simulink model "DC_power"  (R2023a)
settings: Solver=VariableStepAuto  StartTime=0.0  StopTime=5  MaxStep=1e-6  RelTol=1e-3
libraries: fl_lib x11, ee_lib x11, nesl_utility x11, simulink x3, spspowerguiLib x1
settings Model: Creator=MEHMET  LastModifiedBy=MEHMET
settings DebuggingCC: ParameterPrecisionLossMsg=none

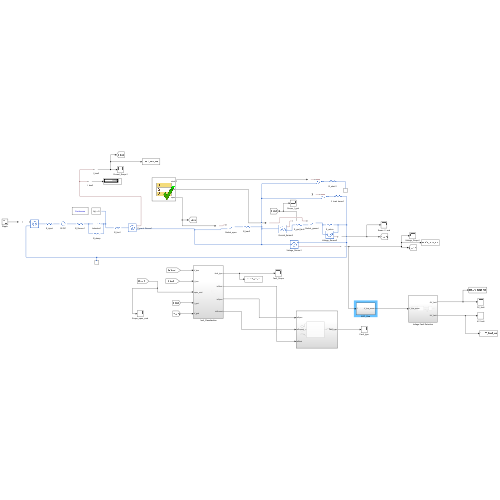
[thumbnail: Simulink's stored preview of the top-level diagram]
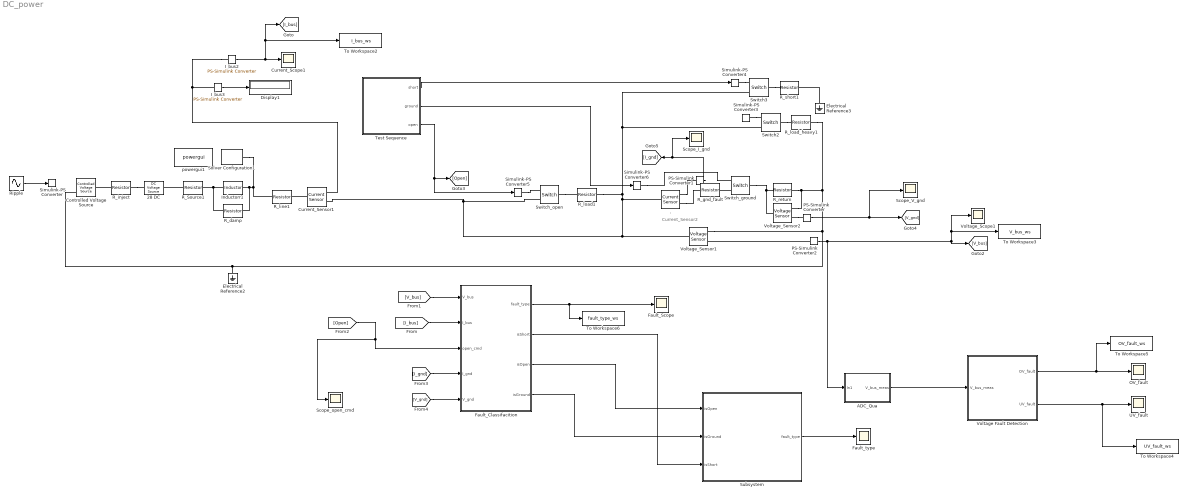
== system DC_power ==
  note: Current_Sensor2
  . : fl_lib/Electrical/Electrical Sensors/Current Sensor
  28 DC : ee_lib/Additional Components/SPICE Sources/DC Voltage Source  DC=28 V
  ADC_Qua : Subsystem
  Controlled Voltage Source : fl_lib/Electrical/Electrical Sources/Controlled Voltage Source
  Current_Scope1 : Scope
  Current_Sensor1 : fl_lib/Electrical/Electrical Sensors/Current Sensor
  Display1 : Display
  Electrical Reference2 : fl_lib/Electrical/Electrical Elements/Electrical Reference
  Electrical Reference3 : fl_lib/Electrical/Electrical Elements/Electrical Reference
  Fault_Classifacition : Subsystem
  Fault_Scope : Scope
  Fault_type : Scope
  I_bus2 : nesl_utility/PS-Simulink Converter  PhysicalDomain=network_engine_domain  SubClassName=ps_output  LeftPortType=input  RightPortType=output  PseudoPeriodic=off  Frequencies=[]  VectorFormat=inherit  Unit=inherit  AffineConversion=off
  I_bus3 : nesl_utility/PS-Simulink Converter  PhysicalDomain=network_engine_domain  SubClassName=ps_output  LeftPortType=input  RightPortType=output  PseudoPeriodic=off  Frequencies=[]  VectorFormat=inherit  Unit=inherit  AffineConversion=off
  Inductorr1 : ee_lib/Passive/Inductor  l=20e-6 H  enable_L_tol=ee.enum.toleranceApplication.none  L_tol=20  tol_distribution=ee.enum.toleranceDistribution.uniform  nSigma=4  r=0 Ohm  g=1e-9 1/Ohm  enable_operating_limits=ee.enum.enable.no  operating_limit_action=ee.enum.passive.reportOpLim.warn  max_working_current=1 A  power_rating=1 W  enable_faults=ee.enum.enable.no  fault_action=simscape.enum.assert.action.none  lambdaPercent=50  k_faulted=0.9999  turnsShort=ee.enum.passive.inductor.turnsShortOption.no  openCct=ee.enum.enable.no  groundShort=ee.enum.passive.inductor.groundShortOption.no  groundShortG=0 1/Ohm  tau_fault=1e-3 s  fault_trigger=ee.enum.faults.faultTrigger.temporal  t_fault=1 s  max_permissible_voltage=100 V  n_fail_on_voltage=1  max_permissible_current=1 A  t_fail_on_current=1 s  i_L_specify=off  i_L_priority=High  i_L=0 A  i_L_nominal_specify=off  i_L_nominal_unit=A  i_L_nominal_value=1
  OV_fault : Scope
  PS-Simulink Converter : nesl_utility/PS-Simulink Converter  PhysicalDomain=network_engine_domain  SubClassName=ps_output  LeftPortType=input  RightPortType=output  PseudoPeriodic=off  Frequencies=[]  VectorFormat=inherit  Unit=inherit  AffineConversion=off
  PS-Simulink Converter1 : nesl_utility/PS-Simulink Converter  PhysicalDomain=network_engine_domain  SubClassName=ps_output  LeftPortType=input  RightPortType=output  PseudoPeriodic=off  Frequencies=[]  VectorFormat=inherit  Unit=inherit  AffineConversion=off
  PS-Simulink Converter2 : nesl_utility/PS-Simulink Converter  PhysicalDomain=network_engine_domain  SubClassName=ps_output  LeftPortType=input  RightPortType=output  PseudoPeriodic=off  Frequencies=[]  VectorFormat=inherit  Unit=inherit  AffineConversion=off
  R_Source1 : ee_lib/Passive/Resistor  R=0.1 Ohm  enable_R_tol=ee.enum.toleranceApplication.none  R_tol=5  tol_distribution=ee.enum.toleranceDistribution.uniform  nSigma=4  enable_operating_limits=ee.enum.enable.no  operating_limit_action=ee.enum.passive.reportOpLim.warn  power_rating=1 W  max_working_voltage=100 V  enable_faults=ee.enum.enable.no  fault_action=simscape.enum.assert.action.none  R_faulted=inf Ohm  fault_trigger=ee.enum.faults.faultTrigger.temporal  t_fault=1 s  max_permissible_current=1 A  t_fail_on_current=1 s  noise_mode=ee.enum.sources.noise.Disabled  Tdevice=25 degC  sample_time=1e-3 s  repeatability=ee.enum.ic.repeatability.notRepeatable  user_seed=0  auto_seed=3890346746  power_derating_T1=70 degC  power_derating_T2=155 degC  operating_temperature_range_vec=[-50, 150] degC  alpha=3.93e-3 1/K  Tmeas=25 degC  thermal_mass=100 J/K  temperature_specify=off  temperature_priority=High  temperature=298.15 K  temperature_nominal_specify=off  temperature_nominal_unit=K  temperature_nominal_value=1
  R_damp : ee_lib/Passive/Resistor  R=10 Ohm  enable_R_tol=ee.enum.toleranceApplication.none  R_tol=5  tol_distribution=ee.enum.toleranceDistribution.uniform  nSigma=4  enable_operating_limits=ee.enum.enable.no  operating_limit_action=ee.enum.passive.reportOpLim.warn  power_rating=1 W  max_working_voltage=100 V  enable_faults=ee.enum.enable.no  fault_action=simscape.enum.assert.action.none  R_faulted=inf Ohm  fault_trigger=ee.enum.faults.faultTrigger.temporal  t_fault=1 s  max_permissible_current=1 A  t_fail_on_current=1 s  noise_mode=ee.enum.sources.noise.Disabled  Tdevice=25 degC  sample_time=1e-3 s  repeatability=ee.enum.ic.repeatability.notRepeatable  user_seed=0  auto_seed=3922919431  power_derating_T1=70 degC  power_derating_T2=155 degC  operating_temperature_range_vec=[-50, 150] degC  alpha=3.93e-3 1/K  Tmeas=25 degC  thermal_mass=100 J/K  temperature_specify=off  temperature_priority=High  temperature=298.15 K  temperature_nominal_specify=off  temperature_nominal_unit=K  temperature_nominal_value=1
  R_gnd_fault : ee_lib/Passive/Resistor  R=5 Ohm  enable_R_tol=ee.enum.toleranceApplication.none  R_tol=5  tol_distribution=ee.enum.toleranceDistribution.uniform  nSigma=4  enable_operating_limits=ee.enum.enable.no  operating_limit_action=ee.enum.passive.reportOpLim.warn  power_rating=1 W  max_working_voltage=100 V  enable_faults=ee.enum.enable.no  fault_action=simscape.enum.assert.action.none  R_faulted=inf Ohm  fault_trigger=ee.enum.faults.faultTrigger.temporal  t_fault=1 s  max_permissible_current=1 A  t_fail_on_current=1 s  noise_mode=ee.enum.sources.noise.Disabled  Tdevice=25 degC  sample_time=1e-3 s  repeatability=ee.enum.ic.repeatability.notRepeatable  user_seed=0  auto_seed=1196140742  power_derating_T1=70 degC  power_derating_T2=155 degC  operating_temperature_range_vec=[-50, 150] degC  alpha=3.93e-3 1/K  Tmeas=25 degC  thermal_mass=100 J/K  temperature_specify=off  temperature_priority=High  temperature=298.15 K  temperature_nominal_specify=off  temperature_nominal_unit=K  temperature_nominal_value=1
  R_inject : ee_lib/Passive/Resistor  R=0.1 Ohm  enable_R_tol=ee.enum.toleranceApplication.none  R_tol=5  tol_distribution=ee.enum.toleranceDistribution.uniform  nSigma=4  enable_operating_limits=ee.enum.enable.no  operating_limit_action=ee.enum.passive.reportOpLim.warn  power_rating=1 W  max_working_voltage=100 V  enable_faults=ee.enum.enable.no  fault_action=simscape.enum.assert.action.none  R_faulted=inf Ohm  fault_trigger=ee.enum.faults.faultTrigger.temporal  t_fault=1 s  max_permissible_current=1 A  t_fail_on_current=1 s  noise_mode=ee.enum.sources.noise.Disabled  Tdevice=25 degC  sample_time=1e-3 s  repeatability=ee.enum.ic.repeatability.notRepeatable  user_seed=0  auto_seed=3499211588  power_derating_T1=70 degC  power_derating_T2=155 degC  operating_temperature_range_vec=[-50, 150] degC  alpha=3.93e-3 1/K  Tmeas=25 degC  thermal_mass=100 J/K  temperature_specify=off  temperature_priority=High  temperature=298.15 K  temperature_nominal_specify=off  temperature_nominal_unit=K  temperature_nominal_value=1
  R_line1 : ee_lib/Passive/Resistor  R=0.2 Ohm  enable_R_tol=ee.enum.toleranceApplication.none  R_tol=5  tol_distribution=ee.enum.toleranceDistribution.uniform  nSigma=4  enable_operating_limits=ee.enum.enable.no  operating_limit_action=ee.enum.passive.reportOpLim.warn  power_rating=1 W  max_working_voltage=100 V  enable_faults=ee.enum.enable.no  fault_action=simscape.enum.assert.action.none  R_faulted=inf Ohm  fault_trigger=ee.enum.faults.faultTrigger.temporal  t_fault=1 s  max_permissible_current=1 A  t_fail_on_current=1 s  noise_mode=ee.enum.sources.noise.Disabled  Tdevice=25 degC  sample_time=1e-3 s  repeatability=ee.enum.ic.repeatability.notRepeatable  user_seed=0  auto_seed=545404223  power_derating_T1=70 degC  power_derating_T2=155 degC  operating_temperature_range_vec=[-50, 150] degC  alpha=3.93e-3 1/K  Tmeas=25 degC  thermal_mass=100 J/K  temperature_specify=off  temperature_priority=High  temperature=298.15 K  temperature_nominal_specify=off  temperature_nominal_unit=K  temperature_nominal_value=1
  R_load1 : ee_lib/Passive/Resistor  R=56 Ohm  enable_R_tol=ee.enum.toleranceApplication.none  R_tol=5  tol_distribution=ee.enum.toleranceDistribution.uniform  nSigma=4  enable_operating_limits=ee.enum.enable.no  operating_limit_action=ee.enum.passive.reportOpLim.warn  power_rating=1 W  max_working_voltage=100 V  enable_faults=ee.enum.enable.no  fault_action=simscape.enum.assert.action.none  R_faulted=inf Ohm  fault_trigger=ee.enum.faults.faultTrigger.temporal  t_fault=1 s  max_permissible_current=1 A  t_fail_on_current=1 s  noise_mode=ee.enum.sources.noise.Disabled  Tdevice=25 degC  sample_time=1e-3 s  repeatability=ee.enum.ic.repeatability.notRepeatable  user_seed=0  auto_seed=3499211588  power_derating_T1=70 degC  power_derating_T2=155 degC  operating_temperature_range_vec=[-50, 150] degC  alpha=3.93e-3 1/K  Tmeas=25 degC  thermal_mass=100 J/K  temperature_specify=off  temperature_priority=High  temperature=298.15 K  temperature_nominal_specify=off  temperature_nominal_unit=K  temperature_nominal_value=1
  R_load_heavy1 : ee_lib/Passive/Resistor  R=14 Ohm  enable_R_tol=ee.enum.toleranceApplication.none  R_tol=5  tol_distribution=ee.enum.toleranceDistribution.uniform  nSigma=4  enable_operating_limits=ee.enum.enable.no  operating_limit_action=ee.enum.passive.reportOpLim.warn  power_rating=1 W  max_working_voltage=100 V  enable_faults=ee.enum.enable.no  fault_action=simscape.enum.assert.action.none  R_faulted=inf Ohm  fault_trigger=ee.enum.faults.faultTrigger.temporal  t_fault=1 s  max_permissible_current=1 A  t_fail_on_current=1 s  noise_mode=ee.enum.sources.noise.Disabled  Tdevice=25 degC  sample_time=1e-3 s  repeatability=ee.enum.ic.repeatability.notRepeatable  user_seed=0  auto_seed=2715962282  power_derating_T1=70 degC  power_derating_T2=155 degC  operating_temperature_range_vec=[-50, 150] degC  alpha=3.93e-3 1/K  Tmeas=25 degC  thermal_mass=100 J/K  temperature_specify=off  temperature_priority=High  temperature=298.15 K  temperature_nominal_specify=off  temperature_nominal_unit=K  temperature_nominal_value=1
  R_return : ee_lib/Passive/Resistor  R=0.05 Ohm  enable_R_tol=ee.enum.toleranceApplication.none  R_tol=5  tol_distribution=ee.enum.toleranceDistribution.uniform  nSigma=4  enable_operating_limits=ee.enum.enable.no  operating_limit_action=ee.enum.passive.reportOpLim.warn  power_rating=1 W  max_working_voltage=100 V  enable_faults=ee.enum.enable.no  fault_action=simscape.enum.assert.action.none  R_faulted=inf Ohm  fault_trigger=ee.enum.faults.faultTrigger.temporal  t_fault=1 s  max_permissible_current=1 A  t_fail_on_current=1 s  noise_mode=ee.enum.sources.noise.Disabled  Tdevice=25 degC  sample_time=1e-3 s  repeatability=ee.enum.ic.repeatability.notRepeatable  user_seed=0  auto_seed=3499211588  power_derating_T1=70 degC  power_derating_T2=155 degC  operating_temperature_range_vec=[-50, 150] degC  alpha=3.93e-3 1/K  Tmeas=25 degC  thermal_mass=100 J/K  temperature_specify=off  temperature_priority=High  temperature=298.15 K  temperature_nominal_specify=off  temperature_nominal_unit=K  temperature_nominal_value=1
  R_short1 : ee_lib/Passive/Resistor  R=0.001 Ohm  enable_R_tol=ee.enum.toleranceApplication.none  R_tol=5  tol_distribution=ee.enum.toleranceDistribution.uniform  nSigma=4  enable_operating_limits=ee.enum.enable.no  operating_limit_action=ee.enum.passive.reportOpLim.warn  power_rating=1 W  max_working_voltage=100 V  enable_faults=ee.enum.enable.no  fault_action=simscape.enum.assert.action.none  R_faulted=inf Ohm  fault_trigger=ee.enum.faults.faultTrigger.temporal  t_fault=1 s  max_permissible_current=1 A  t_fail_on_current=1 s  noise_mode=ee.enum.sources.noise.Disabled  Tdevice=25 degC  sample_time=1e-3 s  repeatability=ee.enum.ic.repeatability.notRepeatable  user_seed=0  auto_seed=418932850  power_derating_T1=70 degC  power_derating_T2=155 degC  operating_temperature_range_vec=[-50, 150] degC  alpha=3.93e-3 1/K  Tmeas=25 degC  thermal_mass=100 J/K  temperature_specify=off  temperature_priority=High  temperature=298.15 K  temperature_nominal_specify=off  temperature_nominal_unit=K  temperature_nominal_value=1
  Ripple : Sin  Amplitude=0.3  Frequency=1000  SampleTime=0
  Scope_I_gnd : Scope
  Scope_V_gnd : Scope
  Scope_open_cmd : Scope
  Simulink-PS Converter{,3..6} (5 alike) : nesl_utility/Simulink-PS Converter  PhysicalDomain=network_engine_domain  SubClassName=ps_input  LeftPortType=input  RightPortType=output  PseudoPeriodic=off  Frequencies=[]  NoiseDistribution=none  NoiseParameters=[]  Unit=1  AffineConversion=off  FilteringAndDerivatives=provide  SimscapeFilterOrder=1  InputFilterTimeConstant=0.001  UdotUserProvided=0
  Solver Configuration1 : nesl_utility/Solver Configuration  PhysicalDomain=network_engine_domain  SubClassName=solver  LeftPortType=input  RightPortType=generic  Tones=[]  Harmonics=[]  SimulateNoise=off  Profile=off  UseLocalSampling=off  EnableSwitchedLinearOptims=on  FrequencyDomain=off  UseCCode=off  RelTol=0.001  AbsTol=0.001  MinStep=1e-09  ToWorkspace=off  RevertToSquareIcSolve=off  NumHomotopyIterations=100  PhasorMode=off  PhasorModeNumHarmonics=1  ConsistencySolver=NEWTON_XTOL_AFTER_FTOL  IndexReductionMethod=DerivativeReplacement  DoDC=off  ResidualTolerance=1e-09  ConsistencyTolSource=GLOBAL  ConsistencyAbsTol=0.001  ConsistencyRelTol=0.001  ConsistencyTolFactor=0.001  UseLocalSolver=off  LocalSolverChoice=NE_BACKWARD_EULER_ADVANCER  ResolveIndetEquations=on  FunctionEvalNumThread=1  LocalSolverSampleTime=0.001  DoFixedCost=off  MaxNonlinIter=3  MaxModeIter=2  ComputeImpulses=off  ImpulseIterations=2  LinearAlgebra=auto  LinearAlgebraNumThread=0  EquationFormulation=NE_TIME_EF  DelaysMemoryBudget=1024  AutomaticFiltering=on  FilteringTimeConstant=0.001  PartitionStorageMethod=AS_NEEDED  PartitionMemoryBudget=1024  PartitionMethod=ROBUST
  Subsystem : Subsystem
  Switch2 : fl_lib/Electrical/Electrical Elements/Switch  R_closed=0.01 Ohm  G_open=1e-8 1/Ohm  Threshold=0.5  i_specify=off  i_priority=None  i=0 A  i_nominal_specify=off  i_nominal_unit=A  i_nominal_value=1  v_specify=off  v_priority=None  v=0 V  v_nominal_specify=off  v_nominal_unit=V  v_nominal_value=1
  Switch3 : fl_lib/Electrical/Electrical Elements/Switch  R_closed=0.01 Ohm  G_open=1e-8 1/Ohm  Threshold=0.5  i_specify=off  i_priority=None  i=0 A  i_nominal_specify=off  i_nominal_unit=A  i_nominal_value=1  v_specify=off  v_priority=None  v=0 V  v_nominal_specify=off  v_nominal_unit=V  v_nominal_value=1
  Switch_ground : fl_lib/Electrical/Electrical Elements/Switch  R_closed=0.01 Ohm  G_open=1e-8 1/Ohm  Threshold=0.5  i_specify=off  i_priority=None  i=0 A  i_nominal_specify=off  i_nominal_unit=A  i_nominal_value=1  v_specify=off  v_priority=None  v=0 V  v_nominal_specify=off  v_nominal_unit=V  v_nominal_value=1
  Switch_open : fl_lib/Electrical/Electrical Elements/Switch  R_closed=0.01 Ohm  G_open=1e-8 1/Ohm  Threshold=0.5  i_specify=off  i_priority=None  i=0 A  i_nominal_specify=off  i_nominal_unit=A  i_nominal_value=1  v_specify=off  v_priority=None  v=0 V  v_nominal_specify=off  v_nominal_unit=V  v_nominal_value=1
  Test Sequence : Test Sequence  TreatAsAtomicUnit=on
  To Workspace2 : ToWorkspace  VariableName=I_bus_ws  SaveFormat=Structure With Time  SampleTime=-1
  To Workspace3 : ToWorkspace  VariableName=V_bus_ws  SaveFormat=Structure With Time  SampleTime=-1
      settings: MaxDataPoints=Inf
  To Workspace4 : ToWorkspace  VariableName=UV_fault_ws  SaveFormat=Timeseries  SampleTime=-1
  To Workspace5 : ToWorkspace  VariableName=OV_fault_ws  SaveFormat=Timeseries  SampleTime=-1
  To Workspace6 : ToWorkspace  VariableName=fault_type_ws  SaveFormat=Timeseries  SampleTime=-1
  UV_fault : Scope
  Voltage Fault Detection : Subsystem
  Voltage_Scope1 : Scope
  Voltage_Sensor1 : fl_lib/Electrical/Electrical Sensors/Voltage Sensor
  Voltage_Sensor2 : fl_lib/Electrical/Electrical Sensors/Voltage Sensor
  powergui1 : spspowerguiLib/powergui  Priority=1  SimulationMode=Continuous  SampleTime=50e-6  frequency=60  Iterations=50  frequencyindice=60  Pbase=100e6  ErrMax=1e-4  UnitsV=kV  UnitsW=MW  buscounter=0  FunctionMessages=off  echomessages=off  EnableUseOfTLC=off  CurrentSourceSwitches=off  DisableSnubberDevices=off  DisableRonSwitches=off  DisableVfSwitches=off  DisplayEquations=off  AutomaticDiscreteSolvers=off  SolverType=Tustin/Backward Euler (TBE)  Interpol=off  ExternalGateDelay=off  methode=off  Ts=100  x0status=blocks  SPID=on  SwTol=0  HookPort=off  NonlinearTolerance=1e-4  nMaxIteration=100  ContinueOnMaxIteration=off  RestoreLinks=warning  ResistiveCurrentMeasurement=off  Frange=[0:2:500]  Ylog=off  Xlog=on  ShowGrid=off  save=off  variable=ZData  structure=0  ZoomFFT=off  StartTime=0.0  cycles=1  DisplayStyle=1  fundamental=60  FreqAxis=off  MaxFrequency=1000  frequencyindicesteady=1  RmsSteady=1  display=off
  wires:
  I_bus3/1 -> Display1/1
  I_bus2/1 -> To Workspace2/1, [I_bus], Current_Scope1/1
  Test Sequence/1(short) -> Simulink-PS Converter4/1
  Test Sequence/2(ground) -> Simulink-PS Converter6/1
  Test Sequence/3(open) -> Simulink-PS Converter5/1, [Open]
  Fault_Classifacition/1(fault_type) -> To Workspace6/1, Fault_Scope/1
  [V_bus] -> Fault_Classifacition/1(V_bus)
  [I_bus] -> Fault_Classifacition/2(I_bus)
  [Open] -> Fault_Classifacition/3(open_cmd), Scope_open_cmd/1
  PS-Simulink Converter/1 -> Scope_V_gnd/1, [V_gnd]
  PS-Simulink Converter1/1 -> Scope_I_gnd/1, [I_gnd]
  [I_gnd] -> Fault_Classifacition/4(I_gnd)
  [V_gnd] -> Fault_Classifacition/5(V_gnd)
  ADC_Qua/1(V_bus_meas) -> Voltage Fault Detection/1(V_bus_meas)
  Voltage Fault Detection/1(OV_fault) -> To Workspace5/1, OV_fault/1
  Fault_Classifacition/3(isOpen) -> Subsystem/1(isOpen)
  Fault_Classifacition/4(isGround) -> Subsystem/2(isGround)
  Fault_Classifacition/2(isShort) -> Subsystem/3(isShort)
  Subsystem/1(fault_type) -> Fault_type/1
  Voltage Fault Detection/2(UV_fault) -> To Workspace4/1, UV_fault/1
  PS-Simulink Converter2/1 -> [V_bus], To Workspace3/1, Voltage_Scope1/1, ADC_Qua/1(In1)
  Ripple/1 -> Simulink-PS Converter/1
  connections:
  R_line1/LConn1 -- Solver Configuration1/RConn1 -- R_damp/RConn1 -- Inductorr1/RConn1
  I_bus2/LConn1 -- Current_Sensor1/RConn1 -- I_bus3/LConn1
  Switch2/LConn1 -- R_load_heavy1/LConn1
  Switch3/LConn1 -- R_short1/LConn1
  Simulink-PS Converter4/RConn1 -- Switch3/RConn1
  Simulink-PS Converter3/RConn1 -- Switch2/RConn1
  Electrical Reference3/LConn1 -- R_short1/RConn1
  PS-Simulink Converter2/LConn1 -- Voltage_Sensor1/RConn1
  Inductorr1/LConn1 -- R_damp/LConn1 -- R_Source1/RConn1
  Current_Sensor1/LConn1 -- R_line1/RConn1
  Voltage_Sensor2/RConn2 -- R_return/RConn1 -- R_load_heavy1/RConn1 -- Electrical Reference2/LConn1 -- Controlled Voltage Source/RConn2 -- Voltage_Sensor1/RConn2
  Voltage_Sensor2/RConn1 -- PS-Simulink Converter/LConn1
  ./RConn1 -- PS-Simulink Converter1/LConn1
  Switch_open/LConn1 -- R_load1/LConn1
  Simulink-PS Converter5/RConn1 -- Switch_open/RConn1
  Voltage_Sensor2/LConn1 -- Switch_ground/LConn1 -- R_return/LConn1
  ./RConn2 -- R_gnd_fault/LConn1
  Simulink-PS Converter6/RConn1 -- Switch_ground/RConn1
  Switch_ground/RConn2 -- R_gnd_fault/RConn1
  R_Source1/LConn1 -- 28 DC/LConn1
  R_inject/RConn1 -- 28 DC/RConn1
  R_inject/LConn1 -- Controlled Voltage Source/LConn1
  Current_Sensor1/RConn2 -- Switch_open/RConn2 -- R_load1/RConn1 -- Switch3/RConn2 -- Switch2/RConn2 -- ./LConn1 -- Voltage_Sensor1/LConn1

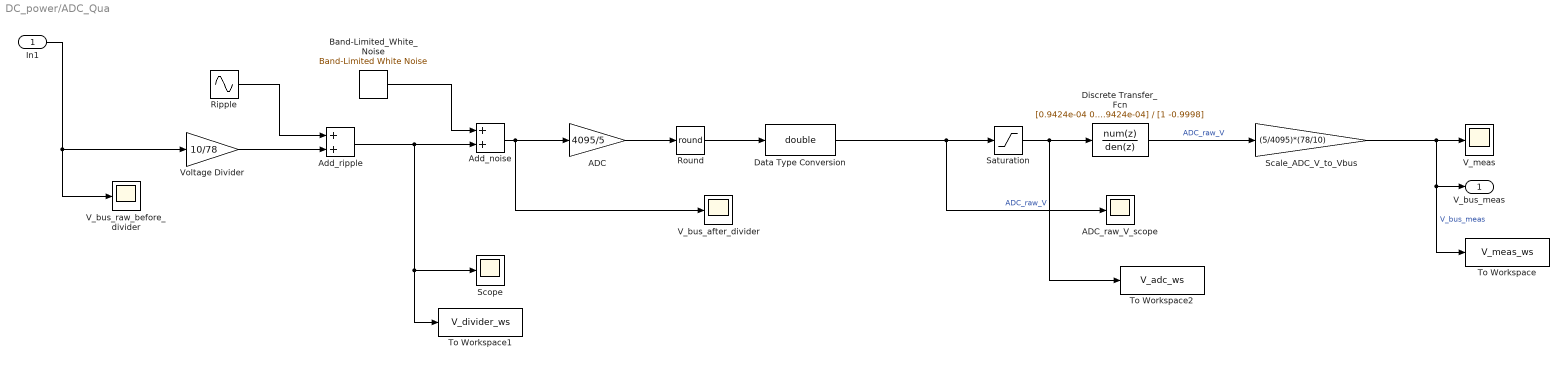
== system DC_power/ADC_Qua ==
  In1 : Inport
  ADC : Gain  Gain=4095/5
  ADC_raw_V_scope : Scope
  Add_noise : Sum
  Add_ripple : Sum
  Band-Limited_White_Noise : simulink/Sources/Band-Limited White Noise  Cov=1e-12  Ts=1e-5  seed=[123]
  Data Type Conversion : DataTypeConversion  OutDataTypeStr=double  SaturateOnIntegerOverflow=off  RndMeth=Floor
  Discrete Transfer_Fcn : DiscreteTransferFcn  Numerator=[0.9424e-04 0.9424e-04]  Denominator=[1 -0.9998]  SampleTime=1e-6
  Ripple : Sin  SampleTime=0
  Round : Rounding  Operator=round
  Saturation : Saturate  UpperLimit=4095  LowerLimit=0  ZeroCross=off
  Scale_ADC_V_to_Vbus : Gain  Gain=(5/4095)*(78/10)
  Scope : Scope
  To Workspace : ToWorkspace  VariableName=V_meas_ws  SaveFormat=Timeseries  SampleTime=-1
  To Workspace1 : ToWorkspace  VariableName=V_divider_ws  SaveFormat=Timeseries  SampleTime=-1
  To Workspace2 : ToWorkspace  VariableName=V_adc_ws  SaveFormat=Timeseries  SampleTime=-1
  V_bus_after_divider : Scope
  V_bus_raw_before_divider : Scope
  V_meas : Scope
  Voltage Divider : Gain  Gain=10/78
  V_bus_meas : Outport
  wires:
  In1/1 -> V_bus_raw_before_divider/1, Voltage Divider/1
  Scale_ADC_V_to_Vbus/1 -> To Workspace/1, V_bus_meas/1, V_meas/1  "V_bus_meas"
  Voltage Divider/1 -> Add_ripple/2
  Add_ripple/1 -> To Workspace1/1, Scope/1, Add_noise/2
  Saturation/1 -> To Workspace2/1, Discrete Transfer_Fcn/1
  Add_noise/1 -> V_bus_after_divider/1, ADC/1
  Round/1 -> Data Type Conversion/1
  Data Type Conversion/1 -> Saturation/1, ADC_raw_V_scope/1  "ADC_raw_V"
  Discrete Transfer_Fcn/1 -> Scale_ADC_V_to_Vbus/1  "ADC_raw_V"
  ADC/1 -> Round/1
  Band-Limited_White_Noise/1 -> Add_noise/1
  Ripple/1 -> Add_ripple/1

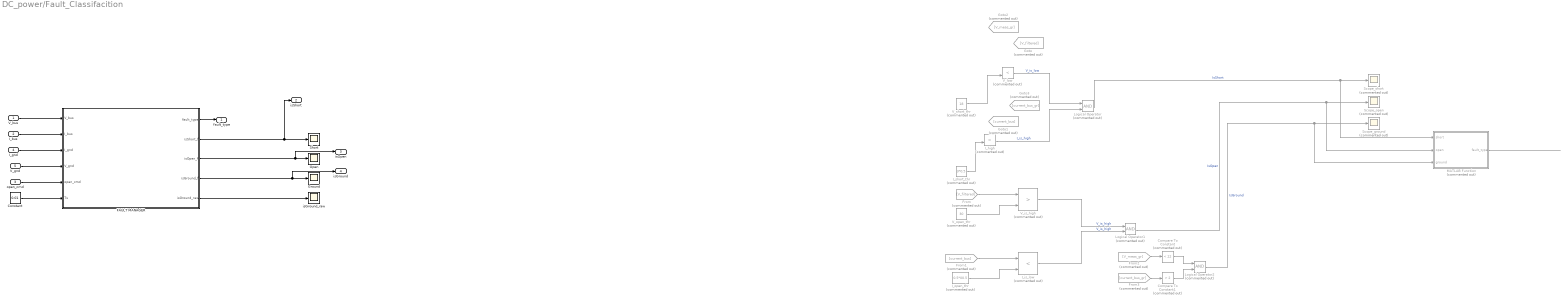
== system DC_power/Fault_Classifacition ==
  V_bus : Inport
  I_bus : Inport  Port=2
  open_cmd : Inport  Port=3
  I_gnd : Inport  Port=4
  V_gnd : Inport  Port=5
  Compare To Constant : simulink/Logic and Bit Operations/Compare To Constant  Commented=on  relop=<  const=22  OutDataTypeStr=boolean  ZeroCross=off
  Compare To Constant1 : simulink/Logic and Bit Operations/Compare To Constant  Commented=on  relop=>  const=2  OutDataTypeStr=boolean  ZeroCross=off
  Constant : Constant  Value=0.01
  FAULT MANAGER : MATLAB Function  TreatAsAtomicUnit=on
  From : From  Commented=on  GotoTag=V_filtered
  From1 : From  Commented=on  GotoTag=current_bus
  From2 : From  Commented=on  GotoTag=V_meas_gr
  From3 : From  Commented=on  GotoTag=current_bus_gr
  Goto : Goto  Commented=on  GotoTag=V_filtered
  Goto1 : Goto  Commented=on  GotoTag=current_bus
  Goto2 : Goto  Commented=on  GotoTag=V_meas_gr
  Goto3 : Goto  Commented=on  GotoTag=current_bus_gr
  Ground : Scope
  I_high : RelationalOperator  Commented=on  Operator=>  OutDataTypeStr=boolean  RndMeth=Simplest  InputSameDT=off
  I_is_low : RelationalOperator  Commented=on  Operator=<  OutDataTypeStr=boolean  RndMeth=Simplest  InputSameDT=off
  I_open_thr : Constant  Commented=on  Value=0.5*00.5
  I_short_thr : Constant  Commented=on  Value=3*0.5
  Logical Operator : Logic  Commented=on  AllPortsSameDT=off  OutDataTypeStr=boolean
  Logical Operator1 : Logic  Commented=on  AllPortsSameDT=off  OutDataTypeStr=boolean
  Logical Operator2 : Logic  Commented=on  AllPortsSameDT=off  OutDataTypeStr=boolean
  MATLAB Function : MATLAB Function  Commented=on  TreatAsAtomicUnit=on
  Open : Scope
  Scope_ground : Scope  Commented=on
  Scope_open : Scope  Commented=on
  Scope_short : Scope  Commented=on
  Short : Scope
  V_is_high : RelationalOperator  Commented=on  Operator=>  OutDataTypeStr=boolean  RndMeth=Simplest  InputSameDT=off
  V_low : RelationalOperator  Commented=on  Operator=<  OutDataTypeStr=boolean  RndMeth=Simplest  InputSameDT=off
  V_open_thr : Constant  Commented=on  Value=30
  V_short_thr : Constant  Commented=on  Value=18
  isGround_raw : Scope
  fault_type : Outport
  isShort : Outport  Port=2
  isOpen : Outport  Port=3
  isGround : Outport  Port=4
  wires:
  ? -> Goto2/1, Goto/1, V_low/1
  V_short_thr/1 -> V_low/2
  V_low/1 -> Logical Operator/1  "V_is_low"
  ? -> Goto3/1, Goto1/1, I_high/1
  I_short_thr/1 -> I_high/2
  I_high/1 -> Logical Operator/2  "I_is_high"
  Logical Operator/1 -> MATLAB Function/1(short), Scope_short/1  "IsShort"
  From/1 -> V_is_high/1
  V_open_thr/1 -> V_is_high/2
  V_is_high/1 -> Logical Operator1/1  "V_is_high"
  I_is_low/1 -> Logical Operator1/2  "V_is_high"
  I_open_thr/1 -> I_is_low/2
  From1/1 -> I_is_low/1
  Logical Operator1/1 -> MATLAB Function/2(open), Scope_open/1  "IsOpen"
  MATLAB Function/1(fault_type) -> ?
  From2/1 -> Compare To Constant/1
  From3/1 -> Compare To Constant1/1
  Compare To Constant/1 -> Logical Operator2/1
  Compare To Constant1/1 -> Logical Operator2/2
  Logical Operator2/1 -> MATLAB Function/3(ground), Scope_ground/1  "IsGround"
  V_bus/1 -> FAULT MANAGER/1(V_bus)
  I_bus/1 -> FAULT MANAGER/2(I_bus)
  Constant/1 -> FAULT MANAGER/6(Ts)
  FAULT MANAGER/2(isShort_f) -> isShort/1, Short/1
  FAULT MANAGER/3(isOpen_f) -> isOpen/1, Open/1
  FAULT MANAGER/4(isGround_f) -> isGround/1, Ground/1
  FAULT MANAGER/1(fault_type) -> fault_type/1
  open_cmd/1 -> FAULT MANAGER/5(open_cmd)
  I_gnd/1 -> FAULT MANAGER/3(I_gnd)
  V_gnd/1 -> FAULT MANAGER/4(V_gnd)
  FAULT MANAGER/5(isGround_raw) -> isGround_raw/1

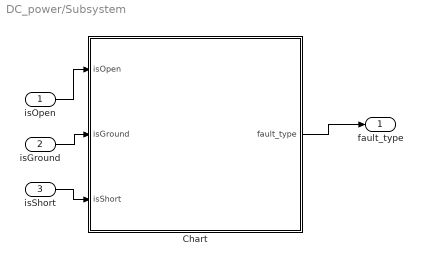
== system DC_power/Subsystem ==
  isOpen : Inport
  isGround : Inport  Port=2
  isShort : Inport  Port=3
  Chart : Stateflow chart  TreatAsAtomicUnit=on
  fault_type : Outport
  wires:
  isShort/1 -> Chart/3(isShort)
  isGround/1 -> Chart/2(isGround)
  isOpen/1 -> Chart/1(isOpen)
  Chart/1(fault_type) -> fault_type/1

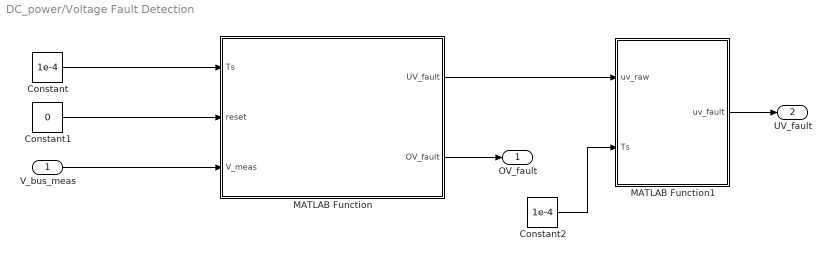
== system DC_power/Voltage Fault Detection ==
  V_bus_meas : Inport
  Constant : Constant  Value=1e-4
  Constant1 : Constant  Value=0
  Constant2 : Constant  Value=1e-4
  MATLAB Function : MATLAB Function  TreatAsAtomicUnit=on
  MATLAB Function1 : MATLAB Function  TreatAsAtomicUnit=on
  OV_fault : Outport
  UV_fault : Outport  Port=2
  wires:
  Constant/1 -> MATLAB Function/1(Ts)
  Constant1/1 -> MATLAB Function/2(reset)
  MATLAB Function/1(UV_fault) -> MATLAB Function1/1(uv_raw)
  MATLAB Function/2(OV_fault) -> OV_fault/1
  Constant2/1 -> MATLAB Function1/2(Ts)
  MATLAB Function1/1(uv_fault) -> UV_fault/1
  V_bus_meas/1 -> MATLAB Function/3(V_meas)

== matlab function DC_power/Fault_Classifacition/FAULT MANAGER ==
  settings: updateMethod=DISCRETE
  data: V_bus input; fault_type output; I_bus input; I_gnd input; V_gnd input; open_cmd input; Ts input; isShort_f output boolean size=1; isOpen_f output boolean size=1; isGround_f output boolean size=1; isGround_raw output boolean size=1
function [fault_type, isShort_f, isOpen_f, isGround_f,isGround_raw] = ...
    fault_manager(V_bus, I_bus,I_gnd, V_gnd, open_cmd, Ts)
% Fault Manager
%  - Short, Open, Ground hatalarını algılar
%  - Debounce (zaman filtresi) uygular
%  - Tek bir fault_type çıktısı üretir
%
% fault_type:
%   0 -> Normal / Heavy
%   1 -> Short
%   2 -> Open
%   3 -> Ground

%% Tunable parametreler (istersen mask parametresi yapabilirsin)
% Short fault eşikleri
V_short_thr  = 18.0;   % V  (bus voltaj çökmesi)
I_short_thr  = 2.0;    % A  (yüksek akım)

% Open fault eşikleri
V_open_thr   = 40.0;   % V  (bus voltajı yüksek)
I_open_thr   = 0.05;   % A  (çok düşük akım)

% Ground fault eşikleri
V_gnd_thr    = 22.0;   % V  (bus gerilimi düşmüş)
I_gnd_thr    = 2.0;    % A  (ground hattında yüksek akım)

% Debounce zamanları (kaç saniye boyunca koşul sağlanmalı?)
debounce_short  = 0.01;   % 10 ms
debounce_open   = 0.01;   % 10 ms
debounce_ground = 0.01;   % 10 ms


%% Persistent sayaçlar (zaman filtresi için)
persistent tShort tOpen tGround
if isempty(tShort)
    tShort  = 0;
    tOpen   = 0;
    tGround = 0;
end

%% 1) RAW FAULT KOŞULLARI
% ----------------------

% Short: Voltaj düşük, akım yüksek
isShort_raw  =(V_bus < V_short_thr) && (I_bus > I_short_thr);

% Open: Sadece open_cmd aktifken kontrol et!
%        => Bu en kritik kısım: test sequence'ten gelen komuta bağlı
isOpen_raw = (open_cmd > 0.5) && (I_bus < I_open_thr);

% Ground: Bus gerilimi düşük, ground hattı akımı yüksek
isGround_raw = (V_gnd < V_gnd_thr)&&(I_gnd > I_gnd_thr);

%% 2) DEBOUNCE / ZAMAN FİLTRESİ
% ----------------------------

% Short timer
if isShort_raw
    tShort = tShort + Ts;
else
    tShort = 0;
end
isShort_f = (tShort >= debounce_short);

% Open timer
if isOpen_raw
    tOpen = tOpen + Ts;
else
    tOpen = 0;
end
isOpen_f = (tOpen >= debounce_open);

% Ground timer
if isGround_raw
    tGround = tGround + Ts;
else
    tGround = 0;
end
isGround_f = (tGround >= debounce_ground);


%% 3) FAULT KLASİFİKASYONU
% ------------------------
% Öncelik: Short > Open > Ground > Normal/Heavy

if isShort_f
    fault_type = uint8(1);   % Short
elseif isOpen_f
    fault_type = uint8(2);   % Open
elseif isGround_f
    fault_type = uint8(3);   % Ground
else
    fault_type = uint8(0);   % Normal / Heavy
end

end

== matlab function DC_power/Fault_Classifacition/MATLAB Function ==
  data: short input; open input; ground input; fault_type output
function fault_type = classify_fault(short, open, ground)

% Gelen sinyalleri net boolean'a çevir
isShort  = (short  > 0.5);
isOpen   = (open   > 0.5);
isGround = (ground > 0.5);

% Öncelik: Short > Open > Ground > Normal
if isShort
    fault_type = uint8(1);   % Short
elseif isOpen
    fault_type = uint8(2);   % Open
elseif isGround
    fault_type = uint8(3);   % Ground
else
    fault_type = uint8(0);   % Normal / Heavy
end
end

== matlab function DC_power/Voltage Fault Detection/MATLAB Function ==
  settings: updateMethod=DISCRETE
  data: UV_fault output; Ts input; reset input; OV_fault output; V_meas input
function [UV_fault, OV_fault] = voltage_fault_detect(Ts, reset, V_meas)

% --- Time base ---
persistent t uv_timer ov_timer
if isempty(t)
    t = 0;
    uv_timer = 0;
    ov_timer = 0;
end

% --- Reset ---
if reset
    t = 0;
    uv_timer = 0;
    ov_timer = 0;
end

% advance time
t = t + Ts;

% --- 704F Mode selection by time (scenario schedule) ---
% Default: Normal operation band
V_UV_TH = 22.0;
V_OV_TH = 29.0;

% --- Detection delays (keep yours) ---
T_UV_DELAY = 0.10;   % s
T_OV_DELAY = 0.05;   % s

% --- Undervoltage logic ---
if V_meas < V_UV_TH
    uv_timer = uv_timer + Ts;
else
    uv_timer = 0;
end

% --- Overvoltage logic ---
if V_meas > V_OV_TH
    ov_timer = ov_timer + Ts;
else
    ov_timer = 0;
end

% --- Fault decision ---
UV_fault = (uv_timer >= T_UV_DELAY);
OV_fault = (ov_timer >= T_OV_DELAY);

end

== stateflow chart DC_power/Test Sequence ==
  state step1
    if t < 2
    % Heavy
    short  = 0;
    open   = 0;
    ground = 0;
    elseif t < 3
    % 1: Short
    short  = 1;
    open   = 0;
    ground = 0;
    elseif t < 4
    % 2: Open
    short  = 0;
    open   = 1;
    ground = 0;
    else
    % 3: Ground
    short  = 0;
    open   = 0;
    ground = 1;
    end
  (default) -> step1
  data: short output double size=1; ground output double size=1; open output size=1

== matlab function DC_power/Voltage Fault Detection/MATLAB Function1 ==
  data: uv_raw input; uv_fault output boolean; Ts input
function uv_fault= UV_Debounce(uv_raw, Ts)

persistent timer
if isempty(timer)
    timer=0;
end

t_confirm= 0.1; % ms debounce

if uv_raw
    timer=timer+Ts;
else
    timer=0;
end

if timer>= t_confirm
    uv_fault=true;
else
    uv_fault=false;
end

== stateflow chart DC_power/Subsystem/Chart ==
  settings: updateMethod=DISCRETE  sampleTime=0.01
  state Short1
    entry:
    fault_type = uint8(1);
  state Normal1
    entry:
    fault_type = uint8(0);
    during:
    if (isShort)  cntShort = cntShort + 1; else cntShort = 0;
    if (isOpen)   cntOpen = cntOpen + 1;  else cntOpen  = 0;
    if (isGround) cntGround = cntGround + 1;else cntGround= 0;
    end
    end
    end
  state Open1
    entry:
    fault_type = uint8(3);
  state Ground1
    entry:
    fault_type = uint8(2);
  Normal1 -> Short1 [order 2] : [ isShort &&cntShort >= N_short&& after(2, tick)]
  Short1 -> Normal1 : [~isShort]
  Normal1 -> Short1 [order 1] : [isShort]
  (default) -> Normal1
  Normal1 -> Ground1 [order 3] : [ isGround && ~isShort && cntGround >= N_ground&&after(3, tick)]
  Normal1 -> Open1 [order 5] : [ isOpen && ~isShort && ~isGround && cntOpen >= N_open &&after(4, tick)]
  Normal1 -> Ground1 [order 6] : [isGround]
  Normal1 -> Open1 [order 4] : [isOpen]
  Ground1 -> Normal1 : [~isGround]
  Open1 -> Normal1 : [~isOpen]
  data: isOpen input boolean size=1; isGround input boolean size=1; fault_type output uint8 size=1; isShort input boolean size=1; cntShort local uint16 size=1 =0; cntOpen local uint16 size=1 =0; cntGround local uint16 size=1 =0; cntUV local uint16 size=1 =0; N_short constant double size=1 =2; N_open constant double size=1 =5; N_ground constant double size=1 =2; N_uv constant double size=1 =10
